simulink subsystem "StudentTemplate"  (R2024b)
settings: Solver=VariableStepAuto  StartTime=0.0  StopTime=10.0  RelTol=1e-3
values from neighbouring files (symbols this model uses):
  circularBufferSize = 25    [runMeFirst.m]
libraries: cstextras x4, cstblocks x3, simulink x2, sldvlib x2, dspswit3 x1
settings Model: Creator=JesseJabezArendse  LastModifiedBy=JesseJabezArendse

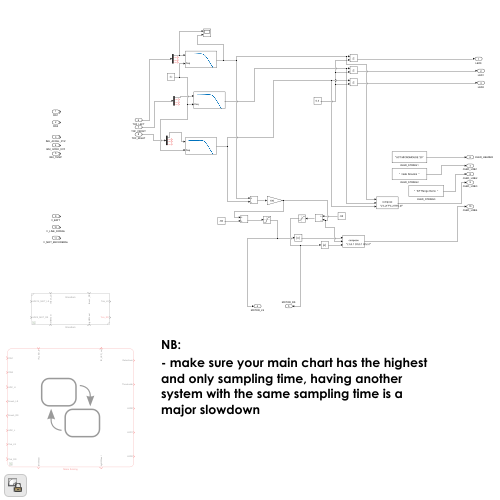
[thumbnail: Simulink's stored preview of the top-level diagram]
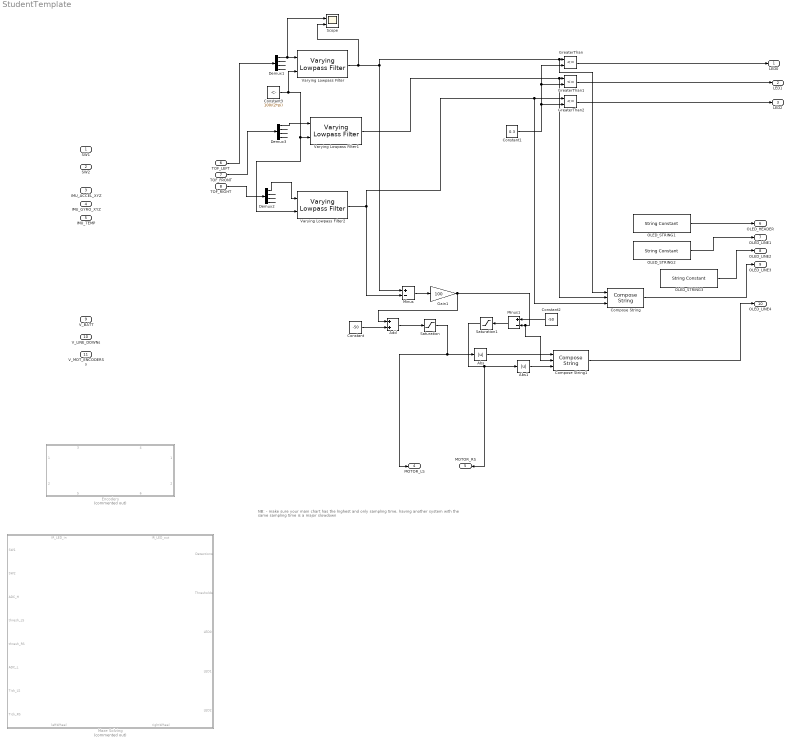
== system StudentTemplate ==
  note: NB:
      |
      | - make sure your main chart has the highest and only sampling time, having another system with the same sampling time is a major slowdown
  SW1 : Inport
  SW2 : Inport  Port=2
  IMU_ACCEL_XYZ : Inport  Port=3
  IMU_GYRO_XYZ : Inport  Port=4
  IMU_TEMP : Inport  Port=5
  TOF_LEFT : Inport  Port=6
  TOF_FRONT : Inport  Port=7
  TOF_RIGHT : Inport  Port=8
  V_BATT : Inport  Port=9
  V_LINE_DOWNs : Inport  Port=10
  V_MOT_ENCODERSs : Inport  Port=11
  Abs : Abs  SaturateOnIntegerOverflow=off
  Abs1 : Abs  SaturateOnIntegerOverflow=off
  Add : Sum
  Compose String : ComposeString  Format="\"L%.2f F%.2f R%.2f\""
  Compose String1 : ComposeString  Format="\"L%3.f  D%3.f  R%3.f\""
  Constant : Constant  Value=-50
  Constant1 : Constant  Value=0.3  SampleTime=-1
  Constant2 : Constant  Value=-50
  Constant3 : Constant  Value=100/(2*pi)
  Demux1 : Demux
  Demux2 : Demux
  Demux3 : Demux
  Encoders : Subsystem  Commented=on  ReferencedSubsystem=Encoders
      settings: PortSchema="{\"entries\":[{\"content\":{\"sides\":[{\"content\":{\"connectorIds\":[\"In1\",\"In2\"]},\"type\":\"ConnectorPlacement.EquallySpacedRectSide\",\"uuid\":\"cd405891-e429-47c4-ab10-86d521705eff\"},{\"content\":{\"connectorIds\":[\"Out1\",\"Out2\"],\"side\":\"RIGHT\"},\"type\":\"ConnectorPlacement.EquallySpacedRectSide\",\"uuid\":\"3a8cc408-692c-4348-91b8-1e484373ad6b\"},{\"content\":{\"connectorIds\":[\"In3\",\"In4\"],\"side\":\"TOP\"},\"type\":\"ConnectorPlacement.EquallySpacedRectSide\",\"uuid\":\"3a691a45-a6f3-4f12-9565-940395609a70\"},{\"content\":{\"connectorIds\":[\"In5\",\"In6\"],\"side\":\"BOTTOM\"},\"type\":\"ConnectorPlacement.EquallySpacedRectSide\",\"uuid\":\"adf6bc66-9d49-4087-b856-4c4b4ba89e7a\"}]},\"type\":\"ConnectorPlacement.EquallySpacedConnector\",\"uuid\":\"1633e398-8e0b-4adb-8010-f61d83ff1f56\"}],\"packageUris\":[\"http://schema.mathworks.com/mf0/Connector/R2020b\"],\"version\":\"1.0\"}"
  Gain1 : Gain  Gain=100
  GreaterThan : RelationalOperator  Operator=<=  OutDataTypeStr=boolean  RndMeth=Simplest  InputSameDT=off
  GreaterThan1 : RelationalOperator  Operator=<=  OutDataTypeStr=boolean  RndMeth=Simplest  InputSameDT=off
  GreaterThan2 : RelationalOperator  Operator=<=  OutDataTypeStr=boolean  RndMeth=Simplest  InputSameDT=off
  Maze Solving : Stateflow chart  Commented=on  TreatAsAtomicUnit=on  SystemSampleTime=0.01
      settings: PortSchema="{\"entries\":[{\"content\":{\"sides\":[{\"content\":{\"connectorIds\":[\"In1\",\"In2\",\"In3\",\"Out9\",\"Out10\",\"In4\",\"In5\",\"In6\"]},\"type\":\"ConnectorPlacement.EquallySpacedRectSide\",\"uuid\":\"32f6fed0-3232-4bab-b39d-a3af84b75639\"},{\"content\":{\"connectorIds\":[\"Out5\",\"Out6\",\"Out1\",\"Out2\",\"Out3\"],\"side\":\"RIGHT\"},\"type\":\"ConnectorPlacement.EquallySpacedRectSide\",\"uuid\":\"0c32a1fe-915a-4e8a-b3ee-800457e23572\"},{\"content\":{\"connectorIds\":[\"In7\",\"Out4\"],\"side\":\"TOP\"},\"type\":\"ConnectorPlacement.EquallySpacedRectSide\",\"uuid\":\"1ac04b60-bb97-4700-a588-8796c93b1b04\"},{\"content\":{\"connectorIds\":[\"Out7\",\"Out8\"],\"side\":\"BOTTOM\"},\"type\":\"ConnectorPlacement.EquallySpacedRectSide\",\"uuid\":\"5382ec1b-aa52-4e38-a7ba-82e952b8f427\"}]},\"type\":\"ConnectorPlacement.EquallySpacedConnector\",\"uuid\":\"e2f36b59-a9e2-4f43-a02a-04bcc2f7ebe2\"}],\"packageUris\":[\"http://schema.mathworks.com/mf0/Connector/R2020b\"],\"version\":\"1.0\"}"
  Minus : Sum  Inputs=+-
  Minus1 : Sum  Inputs=+-
  OLED_STRING1 : StringConstant  String="\"UCT MICROMOUSE '25\""
  OLED_STRING2 : StringConstant  String="\"  Hello Simulink  \""
  OLED_STRING3 : StringConstant  String="\"  ToF Range Demo  \""
  Saturation : Saturate  UpperLimit=100  LowerLimit=-100
  Saturation1 : Saturate  UpperLimit=100  LowerLimit=-100
  Scope : Scope  NumInputPorts=2
  Varying Lowpass Filter : cstblocks/Linear Parameter Varying/Varying Lowpass Filter  N=1
  Varying Lowpass Filter1 : cstblocks/Linear Parameter Varying/Varying Lowpass Filter  N=1
  Varying Lowpass Filter2 : cstblocks/Linear Parameter Varying/Varying Lowpass Filter  N=1
  LED0 : Outport
  LED1 : Outport  Port=2
  LED2 : Outport  Port=3
  MOTOR_LS : Outport  Port=4
  MOTOR_RS : Outport  Port=5
  OLED_HEADER : Outport  Port=6
  OLED_LINE1 : Outport  Port=7
  OLED_LINE2 : Outport  Port=8
  OLED_LINE3 : Outport  Port=9
  OLED_LINE4 : Outport  Port=10
  wires:
  TOF_FRONT/1 -> Demux3/1
  Varying Lowpass Filter2/1 -> Minus/2, GreaterThan2/1, Compose String/3
  Saturation1/1 -> Abs1/1, MOTOR_RS/1
  Varying Lowpass Filter/1 -> GreaterThan/1, Compose String/1, Minus/1, Scope/2
  Minus/1 -> Gain1/1
  OLED_STRING2/1 -> OLED_LINE1/1
  Constant2/1 -> Minus1/1
  Demux2/1 -> Varying Lowpass Filter2/1
  Demux2/3 -> ?
  Demux2/2 -> ?
  Demux2/4 -> ?
  OLED_STRING3/1 -> OLED_LINE2/1
  Varying Lowpass Filter1/1 -> GreaterThan1/1, Compose String/2
  Abs/1 -> Compose String1/1
  GreaterThan1/1 -> LED1/1
  Constant3/1 -> Varying Lowpass Filter/2, Varying Lowpass Filter1/2, Varying Lowpass Filter2/2
  Demux3/3 -> ?
  TOF_RIGHT/1 -> Demux2/1
  Constant/1 -> Add/2
  Compose String1/1 -> OLED_LINE4/1
  Demux3/4 -> ?
  Demux3/2 -> ?
  Demux1/2 -> ?
  Demux3/1 -> Varying Lowpass Filter1/1
  OLED_STRING1/1 -> OLED_HEADER/1
  Abs1/1 -> Compose String1/3
  Demux1/1 -> Varying Lowpass Filter/1, Scope/1
  Minus1/1 -> Saturation1/1
  Compose String/1 -> OLED_LINE3/1
  Constant1/1 -> GreaterThan2/2, GreaterThan1/2, GreaterThan/2
  Saturation/1 -> Abs/1, MOTOR_LS/1
  Demux1/4 -> ?
  GreaterThan2/1 -> LED2/1
  Add/1 -> Saturation/1
  TOF_LEFT/1 -> Demux1/1
  GreaterThan/1 -> LED0/1
  Demux1/3 -> ?
  Gain1/1 -> Add/1, Minus1/2, Compose String1/2

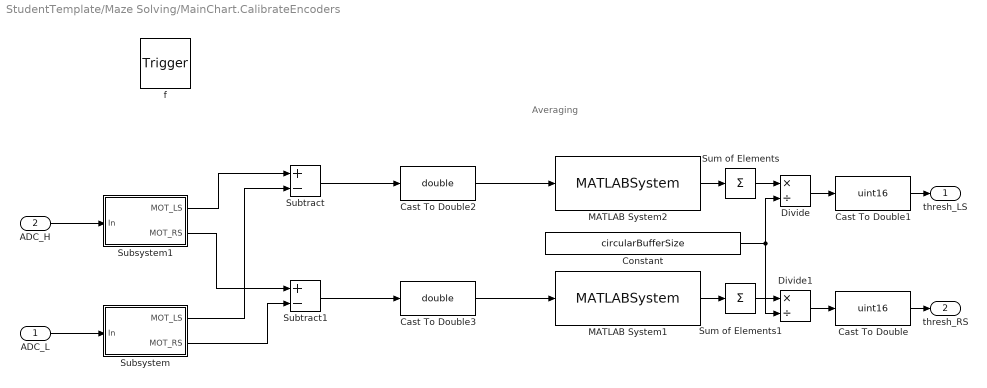
== system StudentTemplate/Maze Solving/MainChart.CalibrateEncoders ==
  note: Averaging
  ADC_L : Inport  OutDataTypeStr=uint16  PortDimensions=8
  ADC_H : Inport  Port=2  OutDataTypeStr=uint16  PortDimensions=8
  f : TriggerPort  TriggerType=function-call  VariantControl=(inherit)
      settings: CopyFcn=Stateflow.SLINSF.SimulinkMan.removeBlockPreDeleteFcn  PreDeleteFcn=Stateflow.SLINSF.SimulinkMan.unsafePredeleteFcn
  Cast To Double : DataTypeConversion  OutDataTypeStr=uint16  SaturateOnIntegerOverflow=off  RndMeth=Floor
  Cast To Double1 : DataTypeConversion  OutDataTypeStr=uint16  SaturateOnIntegerOverflow=off  RndMeth=Floor
  Cast To Double2 : DataTypeConversion  OutDataTypeStr=double  SaturateOnIntegerOverflow=off  RndMeth=Floor
  Cast To Double3 : DataTypeConversion  OutDataTypeStr=double  SaturateOnIntegerOverflow=off  RndMeth=Floor
  Constant : Constant  Value=circularBufferSize  OutDataTypeStr=double
  Divide : Product  Inputs=*/  OutDataTypeStr=Inherit: Same as first input
  Divide1 : Product  Inputs=*/  OutDataTypeStr=Inherit: Same as first input
  MATLAB System1 : MATLABSystem  System=CircularBuffer  BufferLength=circularBufferSize  InitialCondition=0  SimulateUsing=Code generation
      mask Type: CircularBuffer
      mask Display:
      | disp('CircularBuffer');
      | port_label('input',1,'signal');
      | port_label('output',1,'out');
  MATLAB System2 : MATLABSystem  System=CircularBuffer  BufferLength=circularBufferSize  InitialCondition=0  SimulateUsing=Code generation
      mask Type: CircularBuffer
      mask Display:
      | disp('CircularBuffer');
      | port_label('input',1,'signal');
      | port_label('output',1,'out');
  Subsystem : Subsystem
  Subsystem1 : Subsystem
  Subtract : Sum  Inputs=+-
  Subtract1 : Sum  Inputs=+-
  Sum of Elements : Sum  Inputs=+  OutDataTypeStr=Inherit: Same as first input
  Sum of Elements1 : Sum  Inputs=+  OutDataTypeStr=Inherit: Same as first input
  thresh_LS : Outport  OutDataTypeStr=uint16  PortDimensions=1
  thresh_RS : Outport  Port=2  OutDataTypeStr=uint16  PortDimensions=1
  wires:
  ADC_L/1 -> Subsystem/1(In)
  ADC_H/1 -> Subsystem1/1(In)
  Subsystem1/1(MOT_LS) -> Subtract/1
  Subsystem/1(MOT_LS) -> Subtract/2
  Subtract/1 -> Cast To Double2/1
  Subsystem1/2(MOT_RS) -> Subtract1/1
  Subsystem/2(MOT_RS) -> Subtract1/2
  Subtract1/1 -> Cast To Double3/1
  MATLAB System2/1 -> Sum of Elements/1
  MATLAB System1/1 -> Sum of Elements1/1
  Sum of Elements/1 -> Divide/1
  Divide/1 -> Cast To Double1/1
  Sum of Elements1/1 -> Divide1/1
  Divide1/1 -> Cast To Double/1
  Constant/1 -> Divide1/2, Divide/2
  Cast To Double/1 -> thresh_RS/1
  Cast To Double1/1 -> thresh_LS/1
  Cast To Double2/1 -> MATLAB System2/1
  Cast To Double3/1 -> MATLAB System1/1

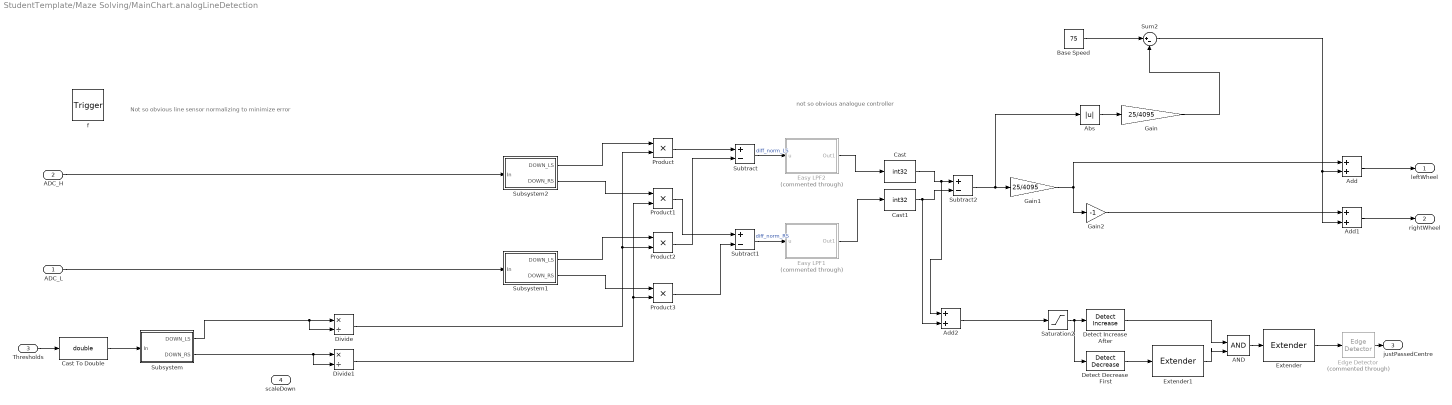
== system StudentTemplate/Maze Solving/MainChart.analogLineDetection ==
  note: Not so obvious line sensor normalizing to minimize error
  note: not so obvious analogue controller
  ADC_L : Inport  OutDataTypeStr=uint16  PortDimensions=8
  ADC_H : Inport  Port=2  OutDataTypeStr=uint16  PortDimensions=8
  Thresholds : Inport  Port=3  OutDataTypeStr=uint16  PortDimensions=8
  scaleDown : Inport  Port=4  OutDataTypeStr=uint16  PortDimensions=1
  f : TriggerPort  TriggerType=function-call  VariantControl=(inherit)
      settings: CopyFcn=Stateflow.SLINSF.SimulinkMan.removeBlockPreDeleteFcn  PreDeleteFcn=Stateflow.SLINSF.SimulinkMan.unsafePredeleteFcn
  AND : Logic  IconShape=distinctive  AllPortsSameDT=off  OutDataTypeStr=boolean
  Abs : Abs  SaturateOnIntegerOverflow=off
  Add : Sum  OutDataTypeStr=int8  AccumDataTypeStr=int8
  Add1 : Sum  OutDataTypeStr=int8  AccumDataTypeStr=int8
  Add2 : Sum
  Base Speed : Constant  Value=75
  Cast : DataTypeConversion  OutDataTypeStr=int32  SaturateOnIntegerOverflow=off  RndMeth=Floor
  Cast To Double : DataTypeConversion  OutDataTypeStr=double  SaturateOnIntegerOverflow=off  RndMeth=Floor
  Cast1 : DataTypeConversion  OutDataTypeStr=int32  SaturateOnIntegerOverflow=off  RndMeth=Floor
  Detect Decrease First : simulink/Logic and Bit Operations/Detect Decrease  vinit=0.0  OutDataTypeStr=boolean
  Detect Increase After : simulink/Logic and Bit Operations/Detect Increase  vinit=0.0  OutDataTypeStr=boolean
  Divide : Product  Inputs=*/
  Divide1 : Product  Inputs=*/
  Easy LPF1 : Subsystem  Commented=through
  Easy LPF2 : Subsystem  Commented=through
  Edge Detector : dspswit3/Edge Detector  Commented=through  InputProcessing=Columns as channels (frame based)
  Extender : sldvlib/Temporal Operators/Extender  reset=off  ext_type=Finite  out_hold=3
  Extender1 : sldvlib/Temporal Operators/Extender  reset=off  ext_type=Finite  out_hold=3
  Gain : Gain  Gain=25/4095
  Gain1 : Gain  Gain=25/4095  OutDataTypeStr=int8
  Gain2 : Gain  Gain=-1
  Product{,1..3} (4 alike) : Product
  Saturation2 : Saturate  UpperLimit=4095*2  LowerLimit=1000
  Subsystem : Subsystem
  Subsystem1 : Subsystem
  Subsystem2 : Subsystem
  Subtract : Sum  Inputs=+-  OutDataTypeStr=int32
  Subtract1 : Sum  Inputs=+-  OutDataTypeStr=int32
  Subtract2 : Sum  Inputs=+-
  Sum2 : Sum  Inputs=|+-
  leftWheel : Outport  OutDataTypeStr=int8  PortDimensions=1
  rightWheel : Outport  Port=2  OutDataTypeStr=int8  PortDimensions=1
  justPassedCentre : Outport  Port=3  OutDataTypeStr=boolean  PortDimensions=1
  wires:
  Thresholds/1 -> Cast To Double/1
  ADC_L/1 -> Subsystem1/1(In)
  ADC_H/1 -> Subsystem2/1(In)
  Subsystem2/1(DOWN_LS) -> Product/1
  Subsystem2/2(DOWN_RS) -> Product1/1
  Subsystem1/1(DOWN_LS) -> Product2/1
  Subsystem1/2(DOWN_RS) -> Product3/1
  Product/1 -> Subtract/1
  Product2/1 -> Subtract/2
  Subtract/1 -> Easy LPF2/1(u)  "diff_norm_LS"
  Product1/1 -> Subtract1/1
  Product3/1 -> Subtract1/2
  Subtract1/1 -> Easy LPF1/1(u)  "diff_norm_RS"
  Add/1 -> leftWheel/1
  Add1/1 -> rightWheel/1
  Subtract2/1 -> Abs/1, Gain1/1
  Sum2/1 -> Add1/2, Add/2
  Cast/1 -> Add2/1, Subtract2/1
  Cast1/1 -> Add2/2, Subtract2/2
  AND/1 -> Extender/1
  Cast To Double/1 -> Subsystem/1(In)
  Subsystem/1(DOWN_LS) -> Divide/2, Divide/1
  Subsystem/2(DOWN_RS) -> Divide1/2, Divide1/1
  Divide/1 -> Product/2, Product2/2
  Divide1/1 -> Product1/2, Product3/2
  Gain1/1 -> Add/1, Gain2/1
  Gain2/1 -> Add1/1
  Base Speed/1 -> Sum2/1
  Abs/1 -> Gain/1
  Gain/1 -> Sum2/2
  Extender/1 -> Edge Detector/1
  Edge Detector/1 -> justPassedCentre/1
  Add2/1 -> Saturation2/1
  Easy LPF2/1(Out1) -> Cast/1
  Easy LPF1/1(Out1) -> Cast1/1
  Saturation2/1 -> Detect Decrease First/1, Detect Increase After/1
  Detect Increase After/1 -> AND/1
  Detect Decrease First/1 -> Extender1/1
  Extender1/1 -> AND/2

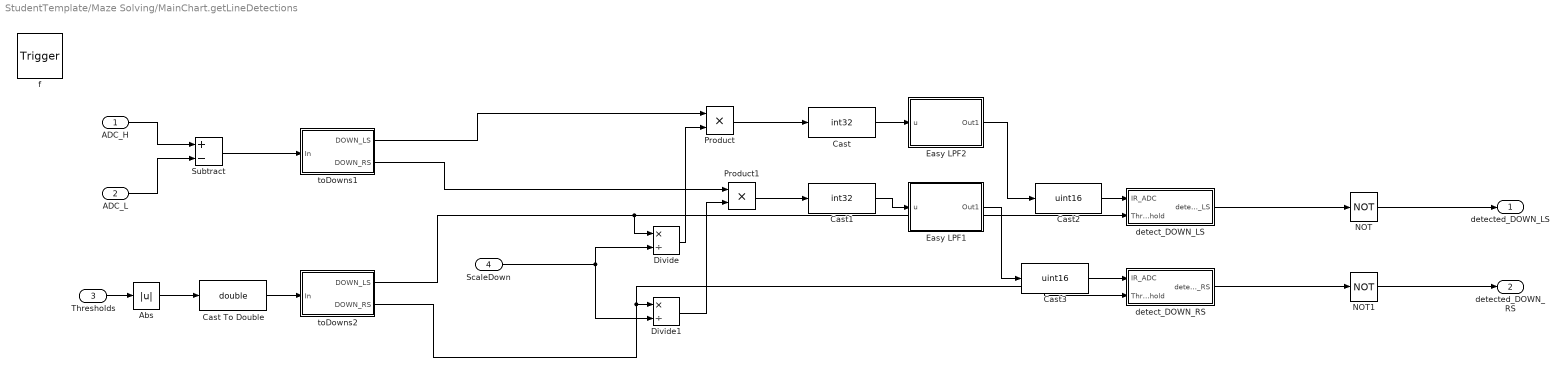
== system StudentTemplate/Maze Solving/MainChart.getLineDetections ==
  ADC_H : Inport  OutDataTypeStr=uint16  PortDimensions=8
  ADC_L : Inport  Port=2  OutDataTypeStr=uint16  PortDimensions=8
  Thresholds : Inport  Port=3  OutDataTypeStr=uint16  PortDimensions=8
  ScaleDown : Inport  Port=4  OutDataTypeStr=uint16  PortDimensions=1
  f : TriggerPort  TriggerType=function-call  VariantControl=(inherit)
      settings: CopyFcn=Stateflow.SLINSF.SimulinkMan.removeBlockPreDeleteFcn  PreDeleteFcn=Stateflow.SLINSF.SimulinkMan.unsafePredeleteFcn
  Abs : Abs  SaturateOnIntegerOverflow=off
  Cast : DataTypeConversion  OutDataTypeStr=int32  SaturateOnIntegerOverflow=off  RndMeth=Floor
  Cast To Double : DataTypeConversion  OutDataTypeStr=double  SaturateOnIntegerOverflow=off  RndMeth=Floor
  Cast1 : DataTypeConversion  OutDataTypeStr=int32  SaturateOnIntegerOverflow=off  RndMeth=Floor
  Cast2 : DataTypeConversion  OutDataTypeStr=uint16  SaturateOnIntegerOverflow=off  RndMeth=Floor
  Cast3 : DataTypeConversion  OutDataTypeStr=uint16  SaturateOnIntegerOverflow=off  RndMeth=Floor
  Divide : Product  Inputs=*/
  Divide1 : Product  Inputs=*/
  Easy LPF1 : Subsystem
  Easy LPF2 : Subsystem
  NOT : Logic  Operator=NOT  IconShape=distinctive  AllPortsSameDT=off  OutDataTypeStr=boolean
  NOT1 : Logic  Operator=NOT  IconShape=distinctive  AllPortsSameDT=off  OutDataTypeStr=boolean
  Product : Product  OutDataTypeStr=uint16
  Product1 : Product  OutDataTypeStr=uint16
  Subtract : Sum  Inputs=+-
  detect_DOWN_LS : Subsystem
  detect_DOWN_RS : Subsystem
  toDowns1 : Subsystem
  toDowns2 : Subsystem
  detected_DOWN_LS : Outport  OutDataTypeStr=boolean  PortDimensions=1
  detected_DOWN_RS : Outport  Port=2  OutDataTypeStr=boolean  PortDimensions=1
  wires:
  Subtract/1 -> toDowns1/1(In)
  Abs/1 -> Cast To Double/1
  NOT/1 -> detected_DOWN_LS/1
  NOT1/1 -> detected_DOWN_RS/1
  Thresholds/1 -> Abs/1
  ADC_L/1 -> Subtract/2
  ADC_H/1 -> Subtract/1
  Product/1 -> Cast/1
  Product1/1 -> Cast1/1
  detect_DOWN_LS/1(detected_DOWN_LS) -> NOT/1
  detect_DOWN_RS/1(detected_DOWN_RS) -> NOT1/1
  toDowns2/2(DOWN_RS) -> detect_DOWN_RS/2(Threshhold), Divide1/1
  toDowns2/1(DOWN_LS) -> Divide/1, detect_DOWN_LS/2(Threshhold)
  toDowns1/1(DOWN_LS) -> Product/1
  toDowns1/2(DOWN_RS) -> Product1/1
  Divide/1 -> Product/2
  Divide1/1 -> Product1/2
  ScaleDown/1 -> Divide/2, Divide1/2
  Cast To Double/1 -> toDowns2/1(In)
  Easy LPF2/1(Out1) -> Cast2/1
  Easy LPF1/1(Out1) -> Cast3/1
  Cast/1 -> Easy LPF2/1(u)
  Cast1/1 -> Easy LPF1/1(u)
  Cast2/1 -> detect_DOWN_LS/1(IR_ADC)
  Cast3/1 -> detect_DOWN_RS/1(IR_ADC)

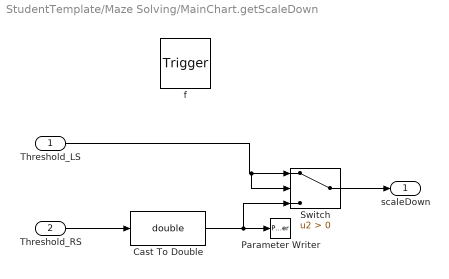
== system StudentTemplate/Maze Solving/MainChart.getScaleDown ==
  Threshold_LS : Inport  OutDataTypeStr=uint16  PortDimensions=1
  Threshold_RS : Inport  Port=2  OutDataTypeStr=uint16  PortDimensions=1
  f : TriggerPort  TriggerType=function-call  VariantControl=(inherit)
      settings: CopyFcn=Stateflow.SLINSF.SimulinkMan.removeBlockPreDeleteFcn  PreDeleteFcn=Stateflow.SLINSF.SimulinkMan.unsafePredeleteFcn
  Cast To Double : DataTypeConversion  OutDataTypeStr=double  SaturateOnIntegerOverflow=off  RndMeth=Floor
  Parameter Writer : ParameterWriter  ParameterOwnerBlock=../Switch  ParameterName=Threshold  ParameterInternalName=Threshold
  Switch : Switch  Criteria=u2 > Threshold  OutDataTypeStr=uint16  SaturateOnIntegerOverflow=off  InputSameDT=off
  scaleDown : Outport  OutDataTypeStr=uint16  PortDimensions=1
  wires:
  Threshold_LS/1 -> Switch/2, Switch/1
  Threshold_RS/1 -> Cast To Double/1
  Switch/1 -> scaleDown/1
  Cast To Double/1 -> Parameter Writer/1, Switch/3

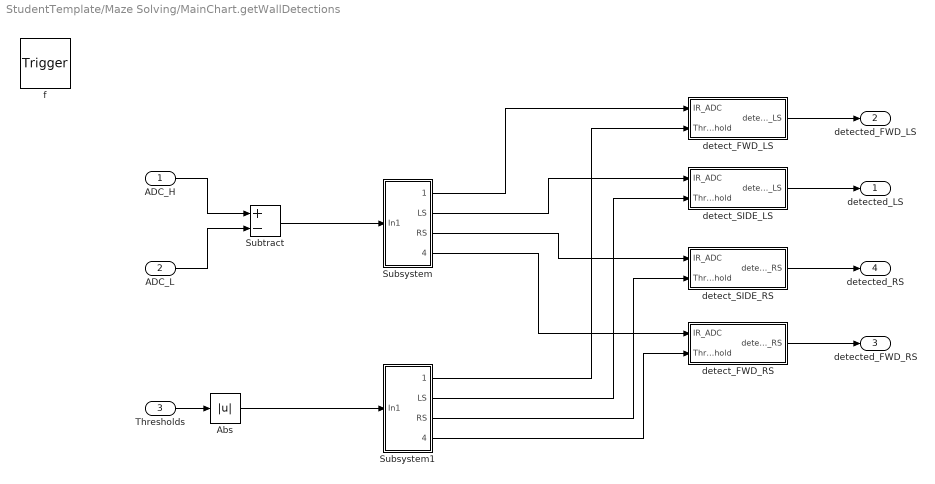
== system StudentTemplate/Maze Solving/MainChart.getWallDetections ==
  ADC_H : Inport  OutDataTypeStr=uint16  PortDimensions=8
  ADC_L : Inport  Port=2  OutDataTypeStr=uint16  PortDimensions=8
  Thresholds : Inport  Port=3  OutDataTypeStr=uint16  PortDimensions=8
  f : TriggerPort  TriggerType=function-call  VariantControl=(inherit)
      settings: CopyFcn=Stateflow.SLINSF.SimulinkMan.removeBlockPreDeleteFcn  PreDeleteFcn=Stateflow.SLINSF.SimulinkMan.unsafePredeleteFcn
  Abs : Abs  SaturateOnIntegerOverflow=off
  Subsystem : Subsystem
  Subsystem1 : Subsystem
  Subtract : Sum  Inputs=+-
  detect_FWD_LS : Subsystem
  detect_FWD_RS : Subsystem
  detect_SIDE_LS : Subsystem
  detect_SIDE_RS : Subsystem
  detected_LS : Outport  OutDataTypeStr=boolean  PortDimensions=1
  detected_FWD_LS : Outport  Port=2  OutDataTypeStr=boolean  PortDimensions=1
  detected_FWD_RS : Outport  Port=3  OutDataTypeStr=boolean  PortDimensions=1
  detected_RS : Outport  Port=4  OutDataTypeStr=boolean  PortDimensions=1
  wires:
  Thresholds/1 -> Abs/1
  ADC_L/1 -> Subtract/2
  ADC_H/1 -> Subtract/1
  detect_FWD_LS/1(detected_FWD_LS) -> detected_FWD_LS/1
  detect_SIDE_LS/1(detected_SIDE_LS) -> detected_LS/1
  detect_SIDE_RS/1(detected_SIDE_RS) -> detected_RS/1
  detect_FWD_RS/1(detected_FWD_RS) -> detected_FWD_RS/1
  Subtract/1 -> Subsystem/1(In1)
  Subsystem/1(FWD_LS) -> detect_FWD_LS/1(IR_ADC)
  Subsystem/2(LS) -> detect_SIDE_LS/1(IR_ADC)
  Subsystem/3(RS) -> detect_SIDE_RS/1(IR_ADC)
  Subsystem/4(FWD_RS) -> detect_FWD_RS/1(IR_ADC)
  Subsystem1/1(FWD_LS) -> detect_FWD_LS/2(Threshhold)
  Subsystem1/2(LS) -> detect_SIDE_LS/2(Threshhold)
  Subsystem1/3(RS) -> detect_SIDE_RS/2(Threshhold)
  Subsystem1/4(FWD_RS) -> detect_FWD_RS/2(Threshhold)
  Abs/1 -> Subsystem1/1(In1)

== system StudentTemplate/Maze Solving/MainChart.CalibrateEncoders/Subsystem ==
  In : Inport  OutDataTypeStr=uint16  PortDimensions=8
  Demux : Demux  Outputs=8
  MOT_LS : Outport
  MOT_RS : Outport  Port=2
  wires:
  Demux/1 -> MOT_LS/1  "MOT_LS"
  Demux/2 -> ?
  Demux/4 -> ?
  Demux/5 -> ?
  In/1 -> Demux/1
  Demux/8 -> MOT_RS/1  "MOT_RS"
  Demux/7 -> ?

== system StudentTemplate/Maze Solving/MainChart.CalibrateEncoders/Subsystem1 ==
  In : Inport  OutDataTypeStr=uint16  PortDimensions=8
  Demux : Demux  Outputs=8
  MOT_LS : Outport
  MOT_RS : Outport  Port=2
  wires:
  Demux/1 -> MOT_LS/1  "MOT_LS"
  Demux/2 -> ?
  Demux/4 -> ?
  Demux/5 -> ?
  In/1 -> Demux/1
  Demux/8 -> MOT_RS/1  "MOT_RS"
  Demux/7 -> ?

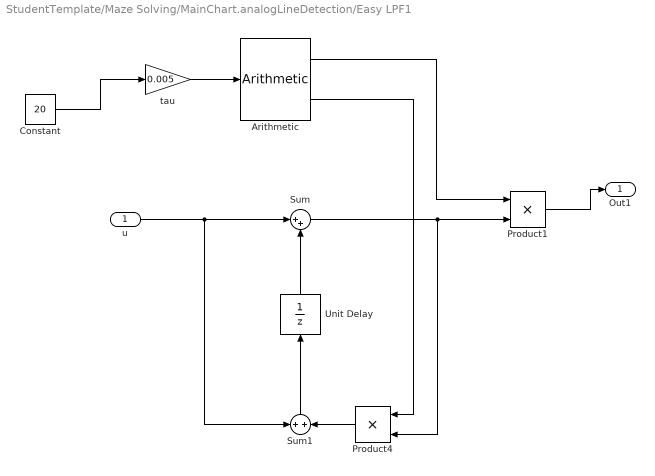
== system StudentTemplate/Maze Solving/MainChart.analogLineDetection/Easy LPF1 ==
  u : Inport
  Arithmetic : cstextras/DiscreteFirstOrderSection/Arithmetic  SystemSampleTime=-1  VariantActivationTime=update diagram  Latency=0  AutoFrameSizeCalculation=off
  Constant : Constant  Value=20
  Product1 : Product
  Product4 : Product
  Sum : Sum  Inputs=|++
  Sum1 : Sum  Inputs=+|+
  Unit Delay : UnitDelay  SampleTime=-1  HasFrameUpgradeWarning=on
  tau : Gain  Tag=#GainSurfaceTarget_  Gain=0.005
  Out1 : Outport
  wires:
  Product1/1 -> Out1/1
  Unit Delay/1 -> Sum/2
  Constant/1 -> tau/1
  Arithmetic/1 -> Product1/1
  u/1 -> Sum/1, Sum1/1
  Sum1/1 -> Unit Delay/1
  Sum/1 -> Product4/2, Product1/2
  Arithmetic/2 -> Product4/1
  tau/1 -> Arithmetic/1
  Product4/1 -> Sum1/2

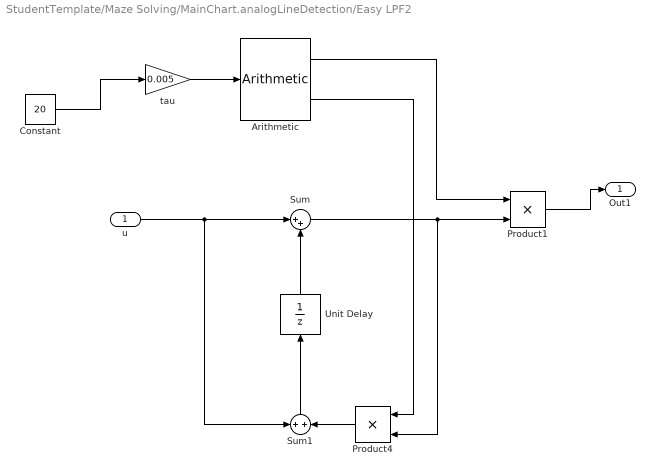
== system StudentTemplate/Maze Solving/MainChart.analogLineDetection/Easy LPF2 ==
  u : Inport
  Arithmetic : cstextras/DiscreteFirstOrderSection/Arithmetic  SystemSampleTime=-1  VariantActivationTime=update diagram  Latency=0  AutoFrameSizeCalculation=off
  Constant : Constant  Value=20
  Product1 : Product
  Product4 : Product
  Sum : Sum  Inputs=|++
  Sum1 : Sum  Inputs=+|+
  Unit Delay : UnitDelay  SampleTime=-1  HasFrameUpgradeWarning=on
  tau : Gain  Tag=#GainSurfaceTarget_  Gain=0.005
  Out1 : Outport
  wires:
  Product1/1 -> Out1/1
  Unit Delay/1 -> Sum/2
  Constant/1 -> tau/1
  Arithmetic/1 -> Product1/1
  u/1 -> Sum/1, Sum1/1
  Sum1/1 -> Unit Delay/1
  Sum/1 -> Product4/2, Product1/2
  Arithmetic/2 -> Product4/1
  tau/1 -> Arithmetic/1
  Product4/1 -> Sum1/2

== system StudentTemplate/Maze Solving/MainChart.analogLineDetection/Subsystem ==
  In : Inport  PortDimensions=8
  Demux : Demux  Outputs=8
  DOWN_LS : Outport
  DOWN_RS : Outport  Port=2
  wires:
  Demux/3 -> DOWN_LS/1  "DOWN_LS"
  Demux/8 -> ?
  Demux/2 -> ?
  Demux/1 -> ?
  Demux/4 -> ?
  Demux/5 -> ?
  In/1 -> Demux/1
  Demux/6 -> DOWN_RS/1  "DOWN_RS"
  Demux/7 -> ?

== system StudentTemplate/Maze Solving/MainChart.analogLineDetection/Subsystem1 ==
  In : Inport  PortDimensions=8
  Demux : Demux  Outputs=8
  DOWN_LS : Outport
  DOWN_RS : Outport  Port=2
  wires:
  Demux/3 -> DOWN_LS/1  "DOWN_LS"
  Demux/8 -> ?
  Demux/2 -> ?
  Demux/1 -> ?
  Demux/4 -> ?
  Demux/5 -> ?
  In/1 -> Demux/1
  Demux/6 -> DOWN_RS/1  "DOWN_RS"
  Demux/7 -> ?

== system StudentTemplate/Maze Solving/MainChart.analogLineDetection/Subsystem2 ==
  In : Inport  PortDimensions=8
  Demux : Demux  Outputs=8
  DOWN_LS : Outport
  DOWN_RS : Outport  Port=2
  wires:
  Demux/3 -> DOWN_LS/1  "DOWN_LS"
  Demux/8 -> ?
  Demux/2 -> ?
  Demux/1 -> ?
  Demux/4 -> ?
  Demux/5 -> ?
  In/1 -> Demux/1
  Demux/6 -> DOWN_RS/1  "DOWN_RS"
  Demux/7 -> ?

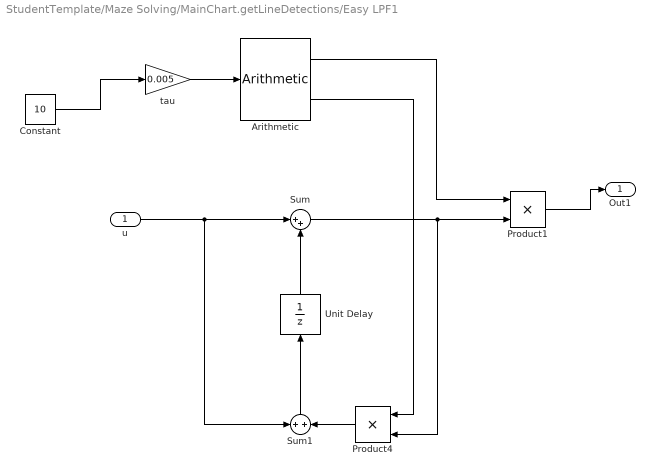
== system StudentTemplate/Maze Solving/MainChart.getLineDetections/Easy LPF1 ==
  u : Inport
  Arithmetic : cstextras/DiscreteFirstOrderSection/Arithmetic  SystemSampleTime=-1  VariantActivationTime=update diagram  AllowFlexibleInterface=on  Latency=0  AutoFrameSizeCalculation=off
  Constant : Constant  Value=10
  Product1 : Product
  Product4 : Product
  Sum : Sum  Inputs=|++
  Sum1 : Sum  Inputs=+|+
  Unit Delay : UnitDelay  SampleTime=-1  HasFrameUpgradeWarning=on
  tau : Gain  Tag=#GainSurfaceTarget_  Gain=0.005
  Out1 : Outport
  wires:
  Product1/1 -> Out1/1
  Unit Delay/1 -> Sum/2
  Constant/1 -> tau/1
  Arithmetic/1 -> Product1/1
  u/1 -> Sum/1, Sum1/1
  Sum1/1 -> Unit Delay/1
  Sum/1 -> Product4/2, Product1/2
  Arithmetic/2 -> Product4/1
  tau/1 -> Arithmetic/1
  Product4/1 -> Sum1/2

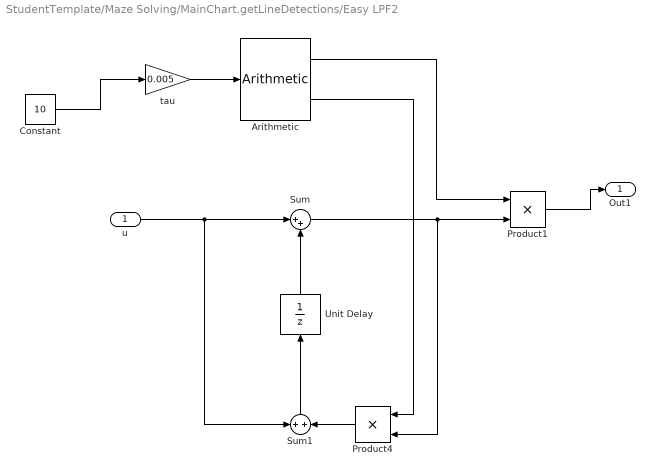
== system StudentTemplate/Maze Solving/MainChart.getLineDetections/Easy LPF2 ==
  u : Inport
  Arithmetic : cstextras/DiscreteFirstOrderSection/Arithmetic  SystemSampleTime=-1  VariantActivationTime=update diagram  AllowFlexibleInterface=on  Latency=0  AutoFrameSizeCalculation=off
  Constant : Constant  Value=10
  Product1 : Product
  Product4 : Product
  Sum : Sum  Inputs=|++
  Sum1 : Sum  Inputs=+|+
  Unit Delay : UnitDelay  SampleTime=-1  HasFrameUpgradeWarning=on
  tau : Gain  Tag=#GainSurfaceTarget_  Gain=0.005
  Out1 : Outport
  wires:
  Product1/1 -> Out1/1
  Unit Delay/1 -> Sum/2
  Constant/1 -> tau/1
  Arithmetic/1 -> Product1/1
  u/1 -> Sum/1, Sum1/1
  Sum1/1 -> Unit Delay/1
  Sum/1 -> Product4/2, Product1/2
  Arithmetic/2 -> Product4/1
  tau/1 -> Arithmetic/1
  Product4/1 -> Sum1/2

== system StudentTemplate/Maze Solving/MainChart.getLineDetections/detect_DOWN_LS ==
  IR_ADC : Inport  OutDataTypeStr=uint16  PortDimensions=1
  Threshhold : Inport  Port=2  PortDimensions=1
  Relational Operator : RelationalOperator  Operator=>  OutDataTypeStr=boolean  RndMeth=Simplest  InputSameDT=off
  detected_DOWN_LS : Outport  OutDataTypeStr=boolean  PortDimensions=1
  wires:
  Relational Operator/1 -> detected_DOWN_LS/1
  Threshhold/1 -> Relational Operator/2
  IR_ADC/1 -> Relational Operator/1

== system StudentTemplate/Maze Solving/MainChart.getLineDetections/detect_DOWN_RS ==
  IR_ADC : Inport  OutDataTypeStr=uint16  PortDimensions=1
  Threshhold : Inport  Port=2  PortDimensions=1
  Relational Operator : RelationalOperator  OutDataTypeStr=boolean  RndMeth=Simplest  InputSameDT=off
  detected_DOWN_RS : Outport  OutDataTypeStr=boolean  PortDimensions=1
  wires:
  Relational Operator/1 -> detected_DOWN_RS/1
  Threshhold/1 -> Relational Operator/2
  IR_ADC/1 -> Relational Operator/1

== system StudentTemplate/Maze Solving/MainChart.getLineDetections/toDowns1 ==
  In : Inport  PortDimensions=8
  Demux : Demux  Outputs=8
  DOWN_LS : Outport  PortDimensions=1
  DOWN_RS : Outport  Port=2  PortDimensions=1
  wires:
  Demux/3 -> DOWN_LS/1  "DOWN_LS"
  Demux/8 -> ?
  Demux/2 -> ?
  Demux/1 -> ?
  Demux/4 -> ?
  Demux/5 -> ?
  In/1 -> Demux/1
  Demux/6 -> DOWN_RS/1  "DOWN_RS"
  Demux/7 -> ?

== system StudentTemplate/Maze Solving/MainChart.getLineDetections/toDowns2 ==
  In : Inport  PortDimensions=8
  Demux : Demux  Outputs=8
  DOWN_LS : Outport  PortDimensions=1
  DOWN_RS : Outport  Port=2  PortDimensions=1
  wires:
  Demux/3 -> DOWN_LS/1  "DOWN_LS"
  Demux/8 -> ?
  Demux/2 -> ?
  Demux/1 -> ?
  Demux/4 -> ?
  Demux/5 -> ?
  In/1 -> Demux/1
  Demux/6 -> DOWN_RS/1  "DOWN_RS"
  Demux/7 -> ?

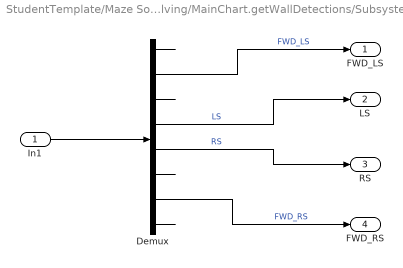
== system StudentTemplate/Maze Solving/MainChart.getWallDetections/Subsystem ==
  In1 : Inport
  Demux : Demux  Outputs=8
  FWD_LS : Outport
  LS : Outport  Port=2
  RS : Outport  Port=3
  FWD_RS : Outport  Port=4
  wires:
  In1/1 -> Demux/1
  Demux/3 -> ?
  Demux/2 -> FWD_LS/1  "FWD_LS"
  Demux/1 -> ?
  Demux/6 -> ?
  Demux/8 -> ?
  Demux/7 -> FWD_RS/1  "FWD_RS"
  Demux/5 -> RS/1  "RS"
  Demux/4 -> LS/1  "LS"

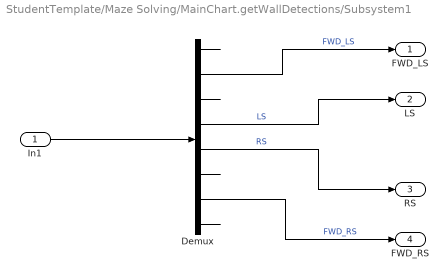
== system StudentTemplate/Maze Solving/MainChart.getWallDetections/Subsystem1 ==
  In1 : Inport  PortDimensions=8
  Demux : Demux  Outputs=8
  FWD_LS : Outport  PortDimensions=1
  LS : Outport  Port=2  PortDimensions=1
  RS : Outport  Port=3  PortDimensions=1
  FWD_RS : Outport  Port=4  PortDimensions=1
  wires:
  Demux/3 -> ?
  Demux/2 -> FWD_LS/1  "FWD_LS"
  Demux/1 -> ?
  Demux/6 -> ?
  Demux/8 -> ?
  Demux/7 -> FWD_RS/1  "FWD_RS"
  Demux/5 -> RS/1  "RS"
  Demux/4 -> LS/1  "LS"
  In1/1 -> Demux/1

== system StudentTemplate/Maze Solving/MainChart.getWallDetections/detect_FWD_LS ==
  IR_ADC : Inport  OutDataTypeStr=uint16  PortDimensions=1
  Threshhold : Inport  Port=2  OutDataTypeStr=uint16  PortDimensions=1
  Relational Operator : RelationalOperator  OutDataTypeStr=boolean  RndMeth=Simplest  InputSameDT=off
  detected_FWD_LS : Outport  OutDataTypeStr=boolean  PortDimensions=1
  wires:
  Relational Operator/1 -> detected_FWD_LS/1
  Threshhold/1 -> Relational Operator/2
  IR_ADC/1 -> Relational Operator/1

== system StudentTemplate/Maze Solving/MainChart.getWallDetections/detect_FWD_RS ==
  IR_ADC : Inport  OutDataTypeStr=uint16  PortDimensions=1
  Threshhold : Inport  Port=2  OutDataTypeStr=uint16  PortDimensions=1
  Relational Operator : RelationalOperator  OutDataTypeStr=boolean  RndMeth=Simplest  InputSameDT=off
  detected_FWD_RS : Outport  OutDataTypeStr=boolean  PortDimensions=1
  wires:
  Relational Operator/1 -> detected_FWD_RS/1
  Threshhold/1 -> Relational Operator/2
  IR_ADC/1 -> Relational Operator/1

== system StudentTemplate/Maze Solving/MainChart.getWallDetections/detect_SIDE_LS ==
  IR_ADC : Inport  OutDataTypeStr=uint16  PortDimensions=1
  Threshhold : Inport  Port=2  OutDataTypeStr=uint16  PortDimensions=1
  Relational Operator : RelationalOperator  OutDataTypeStr=boolean  RndMeth=Simplest  InputSameDT=off
  detected_SIDE_LS : Outport  OutDataTypeStr=boolean  PortDimensions=1
  wires:
  Relational Operator/1 -> detected_SIDE_LS/1
  Threshhold/1 -> Relational Operator/2
  IR_ADC/1 -> Relational Operator/1

== system StudentTemplate/Maze Solving/MainChart.getWallDetections/detect_SIDE_RS ==
  IR_ADC : Inport  OutDataTypeStr=uint16  PortDimensions=1
  Threshhold : Inport  Port=2  OutDataTypeStr=uint16  PortDimensions=1
  Relational Operator : RelationalOperator  OutDataTypeStr=boolean  RndMeth=Simplest  InputSameDT=off
  detected_SIDE_RS : Outport  OutDataTypeStr=boolean  PortDimensions=1
  wires:
  Threshhold/1 -> Relational Operator/2
  IR_ADC/1 -> Relational Operator/1
  Relational Operator/1 -> detected_SIDE_RS/1

== stateflow chart StudentTemplate/Maze Solving ==
  state MainChart
    % you can make chart instance variables like this
    allOff = [false; false; false; false; false; false; false; false];
    during:
    FWD_LS    = Detections(2);
    SIDE_LS    = Detections(4);
    SIDE_RS    = Detections(5);
    FWD_RS    = Detections(7);
    DOWN_LS = Detections(3);
    DOWN_RS = Detections(6);
    state Calibration
      during:
      IR_LED_out = allOff;
      state CalStandby
        during:
        LED0 = ~LED0;
        LED1 = ~LED1;
        LED2 = ~LED2;
        exit:
        LED0 = false;
        LED1 = false;
        LED2 = false;
      state CalWallSensors
        entry:
        IR_LED_out = allOff;
        LED1 = true;
        during:
        IR_LED_out(2) = IR_LED_in(2); % FWD_LS
        IR_LED_out(4) = IR_LED_in(4); % SIDE_LS
        IR_LED_out(5) = IR_LED_in(5); % SIDE_RS
        IR_LED_out(7) = IR_LED_in(7); % FWD_RS
        IR_LED_out(1) = IR_LED_in(1); %MOT_LS
        IR_LED_out(8) = IR_LED_in(8); %MOT_RS
        exit:
        Thresholds(2) = ADC_H(2) - ADC_L(2);
        Thresholds(4) = ADC_H(4) - ADC_L(4);
        Thresholds(5) = ADC_H(5) - ADC_L(5);
        Thresholds(7) = ADC_H(7) - ADC_L(7);
        IR_LED_out = allOff;
      state CalLineSensors
        entry:
        IR_LED_out = allOff;
        LED0 = true;
        during:
        IR_LED_out(3) = IR_LED_in(3); %DOWN_LS
        IR_LED_out(6) = IR_LED_in(6); %DOWN_RS
        exit:
        Thresholds(3) = 2000; %ADC_H(3) - ADC_L(3);%
        Thresholds(6) = 2200; %ADC_H(6) - ADC_L(6);%
        IR_LED_out = allOff;
        [scaleDown] = getScaleDown(Thresholds(3),Thresholds(6));
      state Turn180
        entry:
        leftWheel = 95;
        rightWheel = -95;
        during:
        IR_LED_out(3) = IR_LED_in(3); %DOWN_LS
        IR_LED_out(6) = IR_LED_in(6); %DOWN_RS
        [Detections(3),Detections(6)] = getLineDetections(ADC_H,ADC_L,Thresholds,scaleDown);
        LED0 = Detections(3);
        LED2 = Detections(6);
        LED1 = Detections(3) && Detections(6);
      state CalEncoders
        entry:
        IR_LED_out = allOff;
        LED2 = true;
        leftWheel = -75;
        rightWheel = 75;
        during:
        IR_LED_out(1) = IR_LED_in(1); %MOT_LS
        IR_LED_out(8) = IR_LED_in(8); %MOT_RS
        [thresh_LS,thresh_RS] = CalibrateEncoders(ADC_L,ADC_H);
        exit:
        Thresholds(1) = thresh_LS;
        Thresholds(8) = thresh_RS;
      note: turn 180 then start
      state CalFinish
        entry:
        leftWheel = 75;
        rightWheel = -75;
        during:
        LED0 = ~LED0;
        LED1 = ~LED1;
        LED2 = ~LED2;
        exit:
        leftWheel = 0;
        rightWheel = 0;
      (default) -> CalStandby
      CalStandby -> CalWallSensors : [SW1]
      CalWallSensors -> CalLineSensors : [after(1,sec)]
      CalLineSensors -> Turn180 : after(1,sec)
      CalEncoders -> CalFinish : after(1,sec)
    state MazeFollowing
      entry:
      Thresholds = 0.9 .*Thresholds;
      Thresholds(3) = 0.85*Thresholds(3); %ADC_H(3) - ADC_L(3);%
      Thresholds(6) = 0.85*Thresholds(6); %ADC_H(6) - ADC_L(6);%
      IR_LED_out = allOff;
      during:
      IR_LED_out(1) = IR_LED_in(1); %MOT_LS
      IR_LED_out(8) = IR_LED_in(8); %MOT_RS
      state MakingDecision
        entry:
        LED0 = false;
        LED1 = false;
        LED2 = false;
        during:
        IR_LED_out(3) = IR_LED_in(3); %DOWN_LS
        IR_LED_out(6) = IR_LED_in(6); %DOWN_RS
        [Detections(3),Detections(6)] = getLineDetections(ADC_H,ADC_L,Thresholds,scaleDown);
        exit:
        IR_LED_out = allOff;
        leftWheel = 0;
        rightWheel = 0;
      state DeadEnd
        entry:
        LED0 = true;
        LED1 = false;
        LED2 = true;
        leftWheel = 95;
        rightWheel = -95;
        during:
        LED0 = ~LED0;
        LED1 = ~LED1;
        LED2 = ~LED2;
      state MoveABitForward
        entry:
        leftWheel = 75;
        rightWheel = 75;
      state TurnRight
        during:
        leftWheel = 95;
        rightWheel = -85;
        LED2 = ~LED2;
      state GoStraight
        during:
        leftWheel = 75;
        rightWheel = 75;
        LED1 = ~LED1;
      state TurnLeft
        during:
        leftWheel = -85;
        rightWheel = 95;
        LED0 = ~LED0;
      state StopAndCheckWalls
        entry:
        leftWheel = 0;
        rightWheel = 0;
        during:
        IR_LED_out(2) = IR_LED_in(2); % FWD_LS
        IR_LED_out(4) = IR_LED_in(4); % SIDE_LS
        IR_LED_out(5) = IR_LED_in(5); % SIDE_RS
        IR_LED_out(7) = IR_LED_in(7); % FWD_RS
        [Detections(4),Detections(2),Detections(7),Detections(5)] = getWallDetections(ADC_H,ADC_L,Thresholds);
        LED0 = Detections(4);
        LED1 = Detections(2) && Detections(7);
        LED2 = Detections(5);
        exit:
        %% IR_LED_out = allOff;
      state CatchTheLine
        entry:
        leftWheel = 0;
        rightWheel = 0;
        during:
        IR_LED_out(3) = IR_LED_in(3); %DOWN_LS
        IR_LED_out(6) = IR_LED_in(6); %DOWN_RS
        [leftWheel,rightWheel,justPassedCentre] = analogLineDetection(ADC_L,ADC_H,Thresholds,scaleDown);
        [Detections(3),Detections(6)] = getLineDetections(ADC_H,ADC_L,Thresholds,scaleDown);
        LED0 = Detections(3);
        LED2 = Detections(6);
        LED1 = Detections(3) && Detections(6);
      state FollowUntilCentre
        during:
        IR_LED_out(3) = IR_LED_in(3); %DOWN_LS
        IR_LED_out(6) = IR_LED_in(6); %DOWN_RS
        [leftWheel,rightWheel,justPassedCentre] = analogLineDetection(ADC_L,ADC_H,Thresholds,scaleDown);
        [Detections(3),Detections(6)] = getLineDetections(ADC_H,ADC_L,Thresholds,scaleDown);
        LED0 = Detections(3);
        LED2 = Detections(6);
        LED1 = Detections(3) && Detections(6);
        exit:
        IR_LED_out = allOff;
      MakingDecision -> DeadEnd [order 4] : [FWD_RS && FWD_LS && SIDE_RS && SIDE_LS]
      MoveABitForward -> MakingDecision : [after(0.2,sec)]
      MakingDecision -> TurnLeft [order 3] : [ ~Detections(4)]
      MakingDecision -> CatchTheLine [order 5] : after(1.3,sec)
      MakingDecision -> GoStraight [order 2] : [ (~ Detections(7) || ~ Detections(2))]
      MakingDecision -> TurnRight [order 1] : [ ~Detections(5)]
      StopAndCheckWalls -> MoveABitForward : after(0.8,sec)
      DeadEnd -> CatchTheLine : after(1.2,sec)
      TurnRight -> CatchTheLine : after(0.6,sec)
      TurnLeft -> CatchTheLine : after(0.6,sec)
      GoStraight -> CatchTheLine : after(0.9,sec)
      FollowUntilCentre -> StopAndCheckWalls : [after(3,sec) && justPassedCentre   && (duration(Detections(3) == 1 && Detections(6) == 1) >= 0.5)]
      CatchTheLine -> FollowUntilCentre : [ (DOWN_LS || DOWN_RS)]
      (default) -> FollowUntilCentre
    state [thresh_LS,thresh_RS] = CalibrateEncoders(ADC_L,ADC_H) [function]
    state scaleDown  = getScaleDown(Threshold_LS, Threshold_RS) [function]
    state [detected_LS,detected_FWD_LS,detected_FWD_RS,detected_RS] = getWallDetections(ADC_H,ADC_L,Thresholds) [function]
    state [leftWheel,rightWheel,justPassedCentre] = analogLineDetection(ADC_L,ADC_H,Thresholds,scaleDown) [function]
    state [detected_DOWN_LS,detected_DOWN_RS] = getLineDetections(ADC_H,ADC_L,Thresholds,ScaleDown) [function]
    (default) -> Calibration
    MazeFollowing -> CalStandby : [SW1]
    Turn180 -> MazeFollowing : [after(1.2,sec)]
    CalFinish -> MazeFollowing : after(1,sec)
  (default) -> MainChart
  data: thresh_LS function_output uint16 size=1; thresh_RS function_output uint16 size=1; ADC_L function_input uint16 size=8; ADC_H function_input uint16 size=8; Threshold_LS function_input uint16 size=1; Threshold_RS function_input uint16 size=1; scaleDown function_output uint16 size=1; detected_LS function_output boolean size=1; detected_FWD_LS function_output boolean size=1; detected_FWD_RS function_output boolean size=1; ADC_H function_input uint16 size=8; ADC_L function_input uint16 size=8; Thresholds function_input uint16 size=8; detected_RS function_output boolean size=1; ADC_L function_input uint16 size=8; ADC_H function_input uint16 size=8; Thresholds function_input uint16 size=8; leftWheel function_output int8 size=1; rightWheel function_output int8 size=1; justPassedCentre function_output boolean size=1; scaleDown function_input uint16 size=1; detected_DOWN_LS function_output boolean size=1; detected_DOWN_RS function_output boolean size=1; ADC_H function_input uint16 size=8; ADC_L function_input uint16 size=8; Thresholds function_input uint16 size=8; ScaleDown function_input uint16 size=1; SW1 input boolean size=1; SW2 input boolean size=1; LED0 output boolean size=1 =false; LED1 output boolean size=1 =false; LED2 output boolean size=1 =false; vThreshLower local uint16 size=8; ADC_H input uint16 size=8; ADC_L input uint16 size=8; Tick_LS input uint32 size=1; Tick_RS input uint32 size=1; IR_LED_out output boolean size=8 =[false; false; false; false; false; false; false; false]; vThreshUpper local uint16 size=8; IR_LED_in input boolean size=8; Detections output boolean size=8 =[false; false; false; false; false; false; false; false;]; allOff local boolean size=8; Thresholds output uint16 size=8; leftWheel output int8 size=1; rightWheel output int8 size=1; thresh_LS output uint16 size=1; thresh_RS output uint16 size=1; currTicksL local uint16 size=1 =0; currTicksR local uint16 size=1 =0; justPassedCentre local boolean size=1 =false; DOWN_LS local boolean size=1 =false; DOWN_RS local boolean size=1 =false; FWD_LS local boolean size=1 =false; FWD_RS local boolean size=1 =false; SIDE_LS local boolean size=1 =false; SIDE_RS local boolean size=1 =false; scaleDown local uint16 size=1
